simulink model "check_serial_new_arduino"  (R2020b)
settings: Solver=FixedStepDiscrete  StartTime=0.0  StopTime=inf  FixedStep=0.1  RelTol=1e-3
undefined symbols (not defined in the file or in its folder): Serial_Port, Standard_Devices
libraries: sldrtlib x2
settings Model: Creator=Rahul Subramanian  LastModifiedBy=Rahul Subramanian

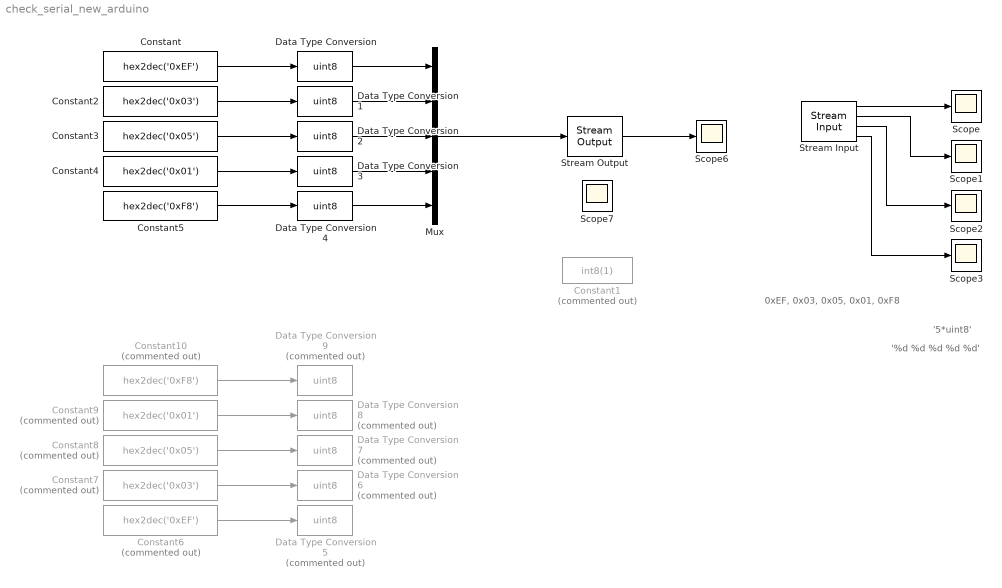
== system check_serial_new_arduino ==
  note: '%d %d %d %d %d'
  note: '5*uint8'
  note: 0xEF, 0x03, 0x05, 0x01, 0xF8
  Constant : Constant  Value=hex2dec('0xEF')
  Constant1 : Constant  Commented=on  Value=int8(1)
  Constant10 : Constant  Commented=on  Value=hex2dec('0xF8')
  Constant2 : Constant  Value=hex2dec('0x03')
  Constant3 : Constant  Value=hex2dec('0x05')
  Constant4 : Constant  Value=hex2dec('0x01')
  Constant5 : Constant  Value=hex2dec('0xF8')
  Constant6 : Constant  Commented=on  Value=hex2dec('0xEF')
  Constant7 : Constant  Commented=on  Value=hex2dec('0x03')
  Constant8 : Constant  Commented=on  Value=hex2dec('0x05')
  Constant9 : Constant  Commented=on  Value=hex2dec('0x01')
  Data Type Conversion{,1..4} (5 alike) : DataTypeConversion  OutDataTypeStr=uint8
  Data Type Conversion{5..9} (5 alike) : DataTypeConversion  Commented=on  OutDataTypeStr=uint8
  Mux : Mux  Inputs=5
  Scope{,1..3,6..7} (6 alike) : Scope
  Stream Input : sldrtlib/Stream Input  SampleTime=0.1  MaxMissedTicks=inf  ShowMissedTicks=on  YieldWhenWaiting=off  DrvName=Standard_Devices/Serial_Port  DrvAddress=5  DrvOptions=[115200 8 0 0 1 0 0 0]  DataTypes='5*uint8'  FormatString='%d %d %d %d %d'  Terminator={'\r \n'}  ShowReady=on  ShowError=on
      settings: AttributesFormatString=Serial Port [5]  SourceProductBaseCode=WT
  Stream Output : sldrtlib/Stream Output  SampleTime=0.1  MaxMissedTicks=inf  ShowMissedTicks=off  YieldWhenWaiting=off  DrvName=Standard_Devices/Serial_Port  DrvAddress=5  DrvOptions=[115200 8 0 0 1 0 0 0]  PortSizes=[5]  FormatString='%d%d%d%d%d'  ShowReady=off  ShowError=on  InitialValue=[]  FinalValue=[]
      settings: AttributesFormatString=Serial Port [5]  SourceProductBaseCode=WT
  wires:
  Stream Input/1 -> Scope/1
  Stream Output/1 -> Scope6/1
  Stream Input/2 -> Scope1/1
  Stream Input/3 -> Scope2/1
  Stream Input/4 -> Scope3/1
  Constant/1 -> Data Type Conversion/1
  Constant2/1 -> Data Type Conversion1/1
  Constant3/1 -> Data Type Conversion2/1
  Constant4/1 -> Data Type Conversion3/1
  Constant5/1 -> Data Type Conversion4/1
  Data Type Conversion/1 -> Mux/1
  Data Type Conversion1/1 -> Mux/2
  Data Type Conversion2/1 -> Mux/3
  Data Type Conversion3/1 -> Mux/4
  Data Type Conversion4/1 -> Mux/5
  Constant10/1 -> Data Type Conversion9/1
  Constant9/1 -> Data Type Conversion8/1
  Constant8/1 -> Data Type Conversion7/1
  Constant7/1 -> Data Type Conversion6/1
  Constant6/1 -> Data Type Conversion5/1
  Mux/1 -> Stream Output/1
